simulink model "control3nema"  (R2025b)
settings: Solver=FixedStepAuto  StartTime=0.0  StopTime=10.0  RelTol=1e-3  EnableMultiTasking=on
undefined symbols (not defined in the file): bits
libraries: stm32f4xxblockslib x6, simulink x4, stm32blockslib x4, svdutilitieslib x2
settings Model: STM32="{\"I2CControllerRead\":[{\"ID\":\"untitled1:33\"},{\"ID\":\"untitled1:86\"},{\"ID\":\"CONTROL2NEMA:33\"},{\"ID\":\"CONTROL2NEMA:86\"}],\"DigitalPortWrite\":[{\"ID\":\"untitled1:37\"},{\"ID\":\"untitled1:38\"},{\"ID\":\"untitled1:90\"},{\"ID\":\"untitled1:91\"},{\"ID\":\"CONTROL2NEMA:37\"},{\"ID\":\"CONTROL2NEMA:38\"},{\"ID\":\"CONTROL2NEMA:90\"},{\"ID\":\"CONTROL2NEMA:91\"}],\"PWMOutput\":[{\"ID\":\"untitled1:39\"},{\"ID\":\"untitled1:92\"},{\"ID\":\"CONTROL2NEMA:39\"},{\"ID\":\"CONTROL2NEMA:92\"}],\"UARTWrite\":[{\"ID\":\"untitled1:47\"},{\"ID\":\"untitled1:100\"},{\"ID\":\"CONTROL2NEMA:47\"},{\"ID\":\"CONTROL2NEMA:100\"}]}"  Creator=hnyur  LastModifiedBy=hnyur
settings OptimizationCC: DefaultParameterBehavior=Inlined  EnhancedBackFolding=on  PassReuseOutputArgsAs=Individual arguments  ZeroExternalMemoryAtStartup=off  ZeroInternalMemoryAtStartup=off  MaxStackSize=512  OptimizeBlockOrder=speed  DifferentSizesBufferReuse=on  OptimizationCustomize=off  EfficientTunableParamExpr=on
settings DebuggingCC: ParameterTunabilityLossMsg=error
settings HardwareCC: ProdBitPerPointer=32.0  ProdBitPerSizeT=32.0  ProdBitPerPtrDiffT=32.0  ProdLargestAtomicInteger=Long  ProdLargestAtomicFloat=Double  ProdWordSize=32.0  ProdLongLongMode=on  ProdHWDeviceType=ARM Compatible->ARM Cortex-M
settings SFSimCC: MATLABDynamicMemAlloc=off
settings RTWCC: SystemTargetFile=ert.tlc  HardwareBoard=STM32H7xx Based (Single-core)  TemplateMakefile=ert_default_tmf  Toolchain=GNU Tools for ARM Embedded Processors  Description=Embedded Coder
settings CodeAppCC: ForceParamTrailComments=on  IgnoreCustomStorageClasses=off  OperatorAnnotations=on  SimulinkDataObjDesc=on  SFDataObjDesc=on  InsertBlockDesc=on
settings ERTTargetCC: ExtModeTransport=3.0  ExtModeStaticAlloc=on  ExtModeStaticAllocSize=2048.0  ExtModeMexFile=ext_xcp  ExtModeIntrfLevel=Level2 - Open  TargetLangStandard=C99 (ISO)  CodeReplacementLibrary=ARM Cortex-M  SupportContinuousTime=on

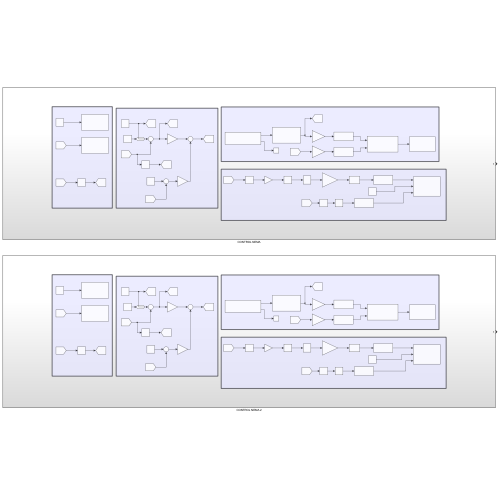
[thumbnail: Simulink's stored preview of the top-level diagram]
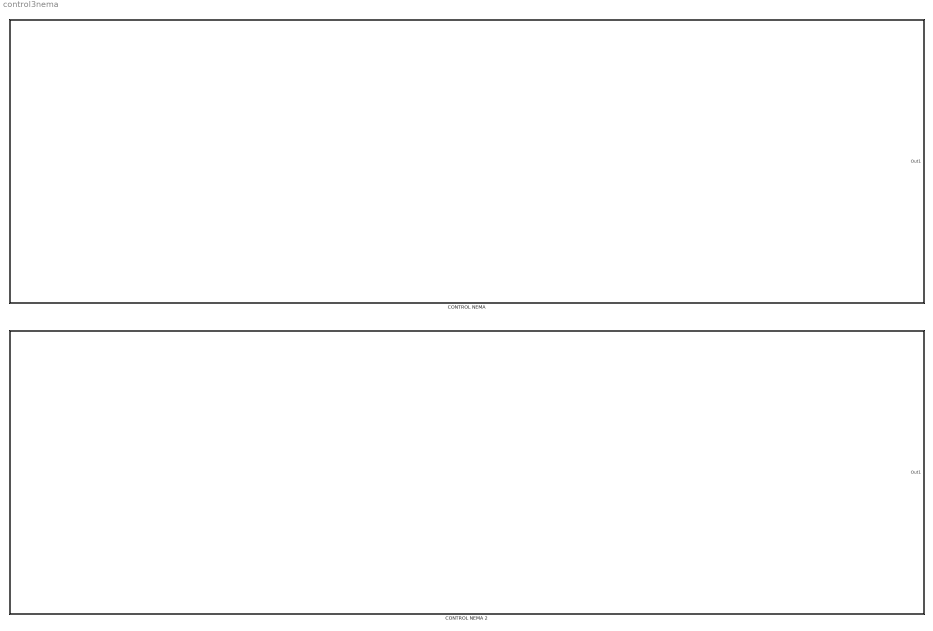
== system control3nema ==
  CONTROL NEMA : Subsystem
  CONTROL NEMA 2 : Subsystem

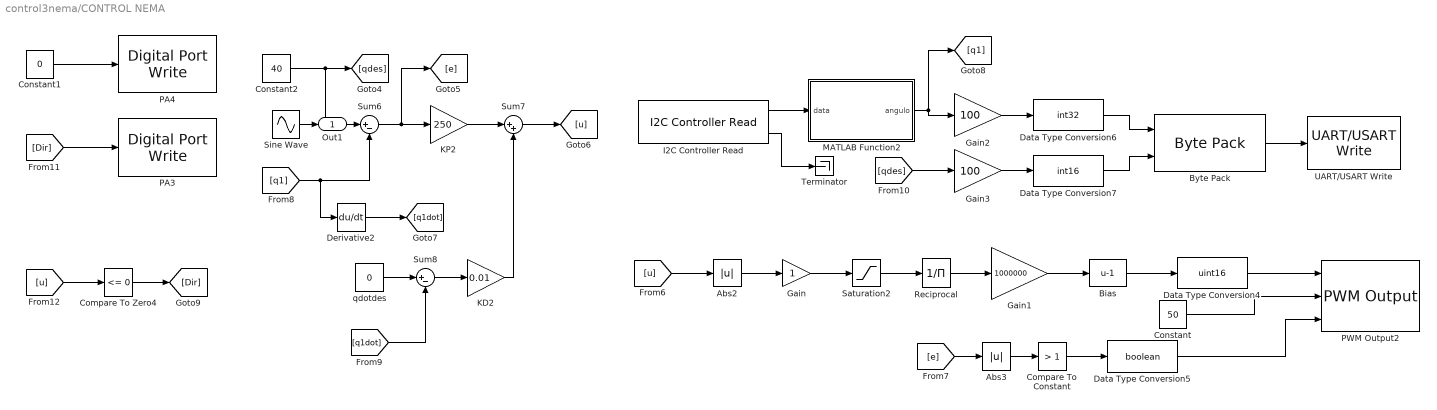
== system control3nema/CONTROL NEMA ==
  Abs2 : Abs  SaturateOnIntegerOverflow=off
  Abs3 : Abs  SaturateOnIntegerOverflow=off
  Bias : Bias  Bias=-1  SaturateOnIntegerOverflow=off
  Byte Pack : svdutilitieslib/Byte Pack  maskPackedDataType=uint8  datatypes={'int32','int16'}  byteAlign=2  blockPlatform=tic2000
      settings: LibrarySourceBlock=c2000lib/Target Communication/Byte Pack
  Compare To Constant : simulink/Logic and Bit Operations/Compare To Constant  relop=>  const=1  OutDataTypeStr=boolean
  Compare To Zero4 : simulink/Logic and Bit Operations/Compare To Zero  relop=<=  OutDataTypeStr=boolean
  Constant : Constant  Value=50
  Constant1 : Constant  Value=0
  Constant2 : Constant  Value=40
  Data Type Conversion4 : DataTypeConversion  OutDataTypeStr=uint16  RndMeth=Floor
  Data Type Conversion5 : DataTypeConversion  OutDataTypeStr=boolean  RndMeth=Floor
  Data Type Conversion6 : DataTypeConversion  OutDataTypeStr=int32  SaturateOnIntegerOverflow=off  RndMeth=Floor
  Data Type Conversion7 : DataTypeConversion  OutDataTypeStr=int16  SaturateOnIntegerOverflow=off  RndMeth=Floor
  Derivative2 : Derivative
  Gain : Gain
  Gain1 : Gain  Gain=1000000
  Gain2 : Gain  Gain=100
  Gain3 : Gain  Gain=100
  I2C Controller Read : stm32blockslib/I2C Controller Read  I2CModule=I2C2  Mode=Controller  AddressingMode=7-bits  PeripheralByteOrder=BigEndian  OwnPeripheralAddress=uint8(170)  PeripheralAddressVia=Dialog  PeripheralAddress=0x36  RegisterAddressMode=on  RegisterAddressVia=Dialog  RegisterAddress=14  RepeatedStart=off  NoAck=off  OutputStatus=on  BlockMode=Receive  DataType=uint8  DataLength=2  Timeout=0.001  SampleTime=0.001
      settings: LibrarySourceBlock=stm32h7xxblockslib/I2C Controller Read
  KD2 : Gain  Gain=0.01
  KP2 : Gain  Gain=250
  MATLAB Function2 : MATLAB Function  TreatAsAtomicUnit=on
  PA3 : stm32f4xxblockslib/Digital Port Write  PortName=GPIOA  PinNumber=3  ReadOperation=off  IOAsArray=on  EnableSimPort=off  hoistedMaskSrc=ECSoC/ECSimCodegen/Digital Port Write
      settings: LibrarySourceBlock=stm32h7xxblockslib/Digital Port Write
  PA4 : stm32f4xxblockslib/Digital Port Write  PortName=GPIOA  PinNumber=4  ReadOperation=off  IOAsArray=on  EnableSimPort=off  hoistedMaskSrc=ECSoC/ECSimCodegen/Digital Port Write
      settings: LibrarySourceBlock=stm32h7xxblockslib/Digital Port Write
  PWM Output2 : stm32f4xxblockslib/PWM Output  ProcessorFamily=STM32G4  TimerModule=TIM13  DutycycleUnits=Counts  EnableChannel1=on  EnableCaptureCompare1Input=off  EnableCaptureCompare1ComplementaryInput=off  EnableOutputCompare1ModeInput=off  EnableChannel2=on  EnableCaptureCompare2Input=off  EnableCaptureCompare2ComplementaryInput=off  EnableOutputCompare2ModeInput=off  EnableChannel3=on  EnableCaptureCompare3Input=off  EnableCaptureCompare3ComplementaryInput=off  EnableOutputCompare3ModeInput=off  EnableChannel4=off  EnableCaptureCompare4Input=off  EnableCaptureCompare4ComplementaryInput=off  EnableOutputCompare4ModeInput=off  EnableChannel5=off  EnableCaptureCompare5Input=off  EnableOutputCompare5ModeInput=off  EnableChannel6=off  EnableCaptureCompare6Input=off  EnableOutputCompare6ModeInput=off  EnableCounterInput=on  EnableMainOutputInput=off  EnableFrequencyInput=on  SetRCAfterCE=off  OutputDirection=off  OutputMainOutputEnableStatus=off  SampleTime=0.1  EnableSimPort=off  EnableUpdateEvent=off  EnableCaptureCompare1Event=off  EnableCaptureCompare2Event=off  EnableCaptureCompare3Event=off  EnableCaptureCompare4Event=off  EnableTriggerEvent=off  EnableBreakEvent=off  EnableBreakEvent2=off  hoistedMaskSrc=ECSoC/ECSimCodegen/PWM Output
      settings: LibrarySourceBlock=stm32h7xxblockslib/PWM Output
  Reciprocal : Product  Inputs=/
  Saturation2 : Saturate  UpperLimit=8000  LowerLimit=1
  Sine Wave : Sin  Amplitude=180  SampleTime=0.001
  Sum6 : Sum  Inputs=|+-
  Sum7 : Sum  Inputs=|++
  Sum8 : Sum  Inputs=|+-
  Terminator : Terminator
  UART/USART Write : stm32blockslib/UART//USART Write  UARTModule=USART3  LengthOfDataToSend=off  BlockingMode=off  BlockingTimeout=0.1  OutputStatus=off
      settings: LibrarySourceBlock=stm32h7xxblockslib/UART//USART Write
  qdotdes : Constant  Value=0
  Out1 : Outport
  wires:
  [Dir] -> PA3/1
  Reciprocal/1 -> Gain1/1
  [e] -> Abs3/1
  [qdes] -> Gain3/1
  Sum7/1 -> [u]
  Constant1/1 -> PA4/1
  KP2/1 -> Sum7/1
  Sine Wave/1 -> Out1/1
  [q1dot] -> Sum8/2
  Abs2/1 -> Gain/1
  Compare To Zero4/1 -> [Dir]
  Saturation2/1 -> Reciprocal/1
  Gain1/1 -> Bias/1
  Bias/1 -> Data Type Conversion4/1
  KD2/1 -> Sum7/2
  Gain/1 -> Saturation2/1
  Compare To Constant/1 -> Data Type Conversion5/1
  Data Type Conversion4/1 -> PWM Output2/1
  Sum6/1 -> [e], KP2/1
  qdotdes/1 -> Sum8/1
  Data Type Conversion6/1 -> Byte Pack/1
  Constant/1 -> PWM Output2/2
  [u] -> Abs2/1
  Gain2/1 -> Data Type Conversion6/1
  [q1] -> Derivative2/1, Sum6/2
  Sum8/1 -> KD2/1
  Gain3/1 -> Data Type Conversion7/1
  Data Type Conversion7/1 -> Byte Pack/2
  MATLAB Function2/1(angulo) -> [q1], Gain2/1
  Byte Pack/1 -> UART/USART Write/1
  I2C Controller Read/1 -> MATLAB Function2/1(data)
  Abs3/1 -> Compare To Constant/1
  [u] -> Compare To Zero4/1
  I2C Controller Read/2 -> Terminator/1
  Constant2/1 -> [qdes], Sum6/1
  Derivative2/1 -> [q1dot]
  Data Type Conversion5/1 -> PWM Output2/3

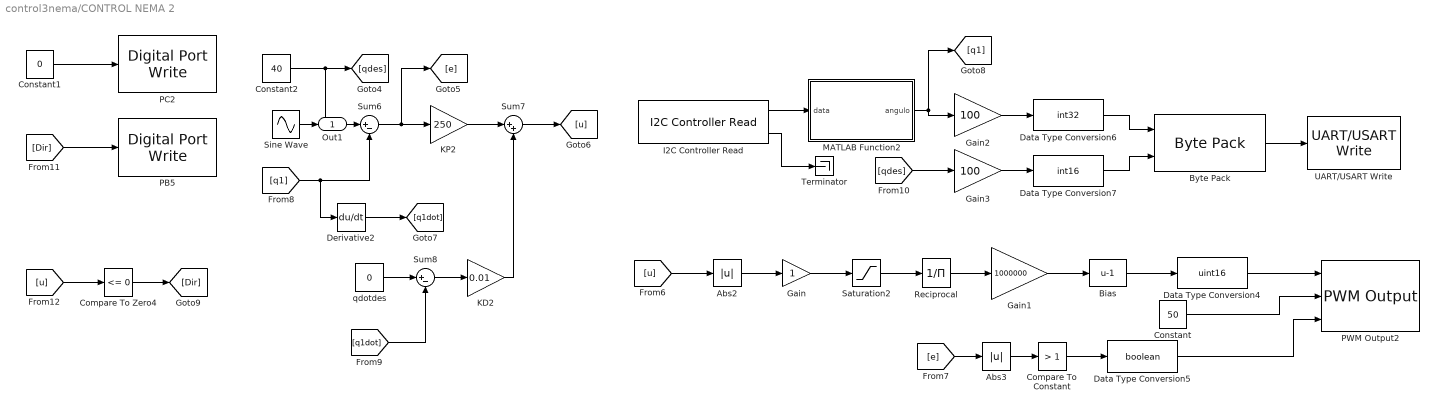
== system control3nema/CONTROL NEMA 2 ==
  Abs2 : Abs  SaturateOnIntegerOverflow=off
  Abs3 : Abs  SaturateOnIntegerOverflow=off
  Bias : Bias  Bias=-1  SaturateOnIntegerOverflow=off
  Byte Pack : svdutilitieslib/Byte Pack  maskPackedDataType=uint8  datatypes={'int32','int16'}  byteAlign=2  blockPlatform=tic2000
      settings: LibrarySourceBlock=c2000lib/Target Communication/Byte Pack
  Compare To Constant : simulink/Logic and Bit Operations/Compare To Constant  relop=>  const=1  OutDataTypeStr=boolean
  Compare To Zero4 : simulink/Logic and Bit Operations/Compare To Zero  relop=<=  OutDataTypeStr=boolean
  Constant : Constant  Value=50
  Constant1 : Constant  Value=0
  Constant2 : Constant  Value=40
  Data Type Conversion4 : DataTypeConversion  OutDataTypeStr=uint16  RndMeth=Floor
  Data Type Conversion5 : DataTypeConversion  OutDataTypeStr=boolean  RndMeth=Floor
  Data Type Conversion6 : DataTypeConversion  OutDataTypeStr=int32  SaturateOnIntegerOverflow=off  RndMeth=Floor
  Data Type Conversion7 : DataTypeConversion  OutDataTypeStr=int16  SaturateOnIntegerOverflow=off  RndMeth=Floor
  Derivative2 : Derivative  CoefficientInTFapproximation=0.001
  Gain : Gain
  Gain1 : Gain  Gain=1000000
  Gain2 : Gain  Gain=100
  Gain3 : Gain  Gain=100
  I2C Controller Read : stm32blockslib/I2C Controller Read  I2CModule=I2C2  Mode=Controller  AddressingMode=7-bits  PeripheralByteOrder=BigEndian  OwnPeripheralAddress=uint8(170)  PeripheralAddressVia=Dialog  PeripheralAddress=0x36  RegisterAddressMode=on  RegisterAddressVia=Dialog  RegisterAddress=14  RepeatedStart=off  NoAck=off  OutputStatus=on  BlockMode=Receive  DataType=uint8  DataLength=2  Timeout=0.001  SampleTime=0.001
      settings: LibrarySourceBlock=stm32h7xxblockslib/I2C Controller Read
  KD2 : Gain  Gain=0.01
  KP2 : Gain  Gain=250
  MATLAB Function2 : MATLAB Function  TreatAsAtomicUnit=on
  PB5 : stm32f4xxblockslib/Digital Port Write  PortName=GPIOA  PinNumber=5  ReadOperation=off  IOAsArray=on  EnableSimPort=off  hoistedMaskSrc=ECSoC/ECSimCodegen/Digital Port Write
      settings: LibrarySourceBlock=stm32h7xxblockslib/Digital Port Write
  PC2 : stm32f4xxblockslib/Digital Port Write  PortName=GPIOA  PinNumber=2  ReadOperation=off  IOAsArray=on  EnableSimPort=off  hoistedMaskSrc=ECSoC/ECSimCodegen/Digital Port Write
      settings: LibrarySourceBlock=stm32h7xxblockslib/Digital Port Write
  PWM Output2 : stm32f4xxblockslib/PWM Output  ProcessorFamily=STM32G4  TimerModule=TIM3  DutycycleUnits=Counts  EnableChannel1=on  EnableCaptureCompare1Input=off  EnableCaptureCompare1ComplementaryInput=off  EnableOutputCompare1ModeInput=off  EnableChannel2=off  EnableCaptureCompare2Input=off  EnableCaptureCompare2ComplementaryInput=off  EnableOutputCompare2ModeInput=off  EnableChannel3=off  EnableCaptureCompare3Input=off  EnableCaptureCompare3ComplementaryInput=off  EnableOutputCompare3ModeInput=off  EnableChannel4=off  EnableCaptureCompare4Input=off  EnableCaptureCompare4ComplementaryInput=off  EnableOutputCompare4ModeInput=off  EnableChannel5=off  EnableCaptureCompare5Input=off  EnableOutputCompare5ModeInput=off  EnableChannel6=off  EnableCaptureCompare6Input=off  EnableOutputCompare6ModeInput=off  EnableCounterInput=on  EnableMainOutputInput=off  EnableFrequencyInput=on  SetRCAfterCE=off  OutputDirection=off  OutputMainOutputEnableStatus=off  SampleTime=0.1  EnableSimPort=off  EnableUpdateEvent=off  EnableCaptureCompare1Event=off  EnableCaptureCompare2Event=off  EnableCaptureCompare3Event=off  EnableCaptureCompare4Event=off  EnableTriggerEvent=off  EnableBreakEvent=off  EnableBreakEvent2=off  hoistedMaskSrc=ECSoC/ECSimCodegen/PWM Output
      settings: LibrarySourceBlock=stm32h7xxblockslib/PWM Output
  Reciprocal : Product  Inputs=/
  Saturation2 : Saturate  UpperLimit=8000  LowerLimit=1
  Sine Wave : Sin  Amplitude=180  SampleTime=0.001
  Sum6 : Sum  Inputs=|+-
  Sum7 : Sum  Inputs=|++
  Sum8 : Sum  Inputs=|+-
  Terminator : Terminator
  UART/USART Write : stm32blockslib/UART//USART Write  UARTModule=USART3  LengthOfDataToSend=off  BlockingMode=off  BlockingTimeout=0.1  OutputStatus=off
      settings: LibrarySourceBlock=stm32h7xxblockslib/UART//USART Write
  qdotdes : Constant  Value=0
  Out1 : Outport
  wires:
  [Dir] -> PB5/1
  Reciprocal/1 -> Gain1/1
  [e] -> Abs3/1
  [qdes] -> Gain3/1
  Sum7/1 -> [u]
  Constant1/1 -> PC2/1
  KP2/1 -> Sum7/1
  Sine Wave/1 -> Out1/1
  [q1dot] -> Sum8/2
  Abs2/1 -> Gain/1
  Compare To Zero4/1 -> [Dir]
  Saturation2/1 -> Reciprocal/1
  Gain1/1 -> Bias/1
  Bias/1 -> Data Type Conversion4/1
  KD2/1 -> Sum7/2
  Gain/1 -> Saturation2/1
  Compare To Constant/1 -> Data Type Conversion5/1
  Data Type Conversion4/1 -> PWM Output2/1
  Sum6/1 -> [e], KP2/1
  qdotdes/1 -> Sum8/1
  Data Type Conversion6/1 -> Byte Pack/1
  Constant/1 -> PWM Output2/2
  [u] -> Abs2/1
  Gain2/1 -> Data Type Conversion6/1
  [q1] -> Derivative2/1, Sum6/2
  Sum8/1 -> KD2/1
  Gain3/1 -> Data Type Conversion7/1
  Data Type Conversion7/1 -> Byte Pack/2
  MATLAB Function2/1(angulo) -> [q1], Gain2/1
  Byte Pack/1 -> UART/USART Write/1
  I2C Controller Read/1 -> MATLAB Function2/1(data)
  Abs3/1 -> Compare To Constant/1
  [u] -> Compare To Zero4/1
  I2C Controller Read/2 -> Terminator/1
  Constant2/1 -> [qdes], Sum6/1
  Derivative2/1 -> [q1dot]
  Data Type Conversion5/1 -> PWM Output2/3

== matlab function control3nema/CONTROL NEMA/MATLAB Function2 ==
  data: data input; angulo output
function angulo = leer_AS5600(data)
% Variables persistentes:
% angulo_anterior almacena la ultima lectura del sensor.
% posicion acumula la posicion angular relativa.
persistent angulo_anterior posicion
% Separar los dos bytes recibidos mediante I2C.
byte_alto = uint16(data(1));
byte_bajo = uint16(data(2));
% Reconstruir el valor de 12 bits del encoder.
conteo = bitor(bitshift(byte_alto,8), byte_bajo);
% Eliminar los cuatro bits que no contienen informacion.
conteo = bitand(conteo,uint16(4095));
% Convertir el conteo a grados.
angulo_actual = double(conteo)*360.0/4096.0;

% Inicializacion de las variables persistentes.
if isempty(angulo_anterior)
angulo_anterior = angulo_actual;
posicion = 0.0;
end
% Calcular el desplazamiento angular entre muestras.
delta = angulo_actual- angulo_anterior;
% Corregir el cambio entre 359 grados y 0 grados.
if delta > 180.0
delta = delta- 360.0;
elseif delta <-180.0
delta = delta + 360.0;
end
% Acumular la posicion relativa.
posicion = posicion + delta;
% Actualizar la lectura anterior.
angulo_anterior = angulo_actual;
% Devolver la posicion angular.
angulo = posicion;
end

== matlab function control3nema/CONTROL NEMA 2/MATLAB Function2 ==
  data: data input; angulo output
function angulo = leer_AS5600(data)
% Variables persistentes:
% angulo_anterior almacena la ultima lectura del sensor.
% posicion acumula la posicion angular relativa.
persistent angulo_anterior posicion
% Separar los dos bytes recibidos mediante I2C.
byte_alto = uint16(data(1));
byte_bajo = uint16(data(2));
% Reconstruir el valor de 12 bits del encoder.
conteo = bitor(bitshift(byte_alto,8), byte_bajo);
% Eliminar los cuatro bits que no contienen informacion.
conteo = bitand(conteo,uint16(4095));
% Convertir el conteo a grados.
angulo_actual = double(conteo)*360.0/4096.0;

% Inicializacion de las variables persistentes.
if isempty(angulo_anterior)
angulo_anterior = angulo_actual;
posicion = 0.0;
end
% Calcular el desplazamiento angular entre muestras.
delta = angulo_actual- angulo_anterior;
% Corregir el cambio entre 359 grados y 0 grados.
if delta > 180.0
delta = delta- 360.0;
elseif delta <-180.0
delta = delta + 360.0;
end
% Acumular la posicion relativa.
posicion = posicion + delta;
% Actualizar la lectura anterior.
angulo_anterior = angulo_actual;
% Devolver la posicion angular.
angulo = posicion;
end
